simulink library "simulink"  (R2014a)
settings: Solver=ode45  SolverMode=SingleTasking  StartTime=0.0  StopTime=10.0  RelTol=1e-3
PostLoadFcn:
  | setsysloc_simulink(bdroot)
undefined symbols (not defined in the file or in its folder): DiscIntNeverNeededParam, getdatatypespecs, NumBits1, NumBits2, sfunxy, sigbuilder_block, slcm, SlDemoSign, Slope1, Slope2
libraries: simulink x40, sl_helperblocks x2, eml_lib x1
(part 5 of 5)

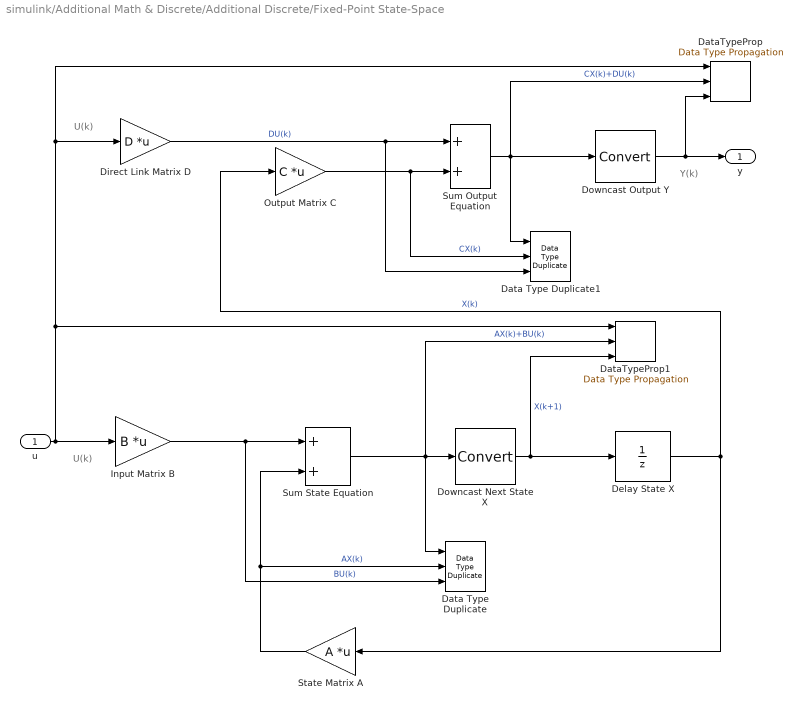
== system simulink/Additional Math & Discrete/Additional Discrete/Fixed-Point State-Space ==
  note: U(k)
  note: U(k)
  note: Y(k)
  u : Inport
  Data Type Duplicate : DataTypeDuplicate  DisableCoverage=on  NumInputPorts=3
  Data Type Duplicate1 : DataTypeDuplicate  DisableCoverage=on  NumInputPorts=3
  DataTypeProp : simulink/Signal Attributes/Data Type Propagation  PropDataType=fixdt(1, 16)  IfRefDouble=double  IfRefSingle=single  IsSigned=IsSigned1 or IsSigned2  NumBitsBase=NumBits1  NumBitsMult=1  NumBitsAdd=0  NumBitsAllowFinal=1:128  PropScaling=2^-10  ValuesUsedBestPrec=[5 -7]  SlopeBase=PosRange2  SlopeMult=1  SlopeAdd=0  BiasBase=Bias2  BiasMult=1  BiasAdd=0
  DataTypeProp1 : simulink/Signal Attributes/Data Type Propagation  PropDataType=fixdt(1, 16)  IfRefDouble=double  IfRefSingle=single  IsSigned=IsSigned1 or IsSigned2  NumBitsBase=NumBits1  NumBitsMult=1  NumBitsAdd=0  NumBitsAllowFinal=1:128  PropScaling=2^-10  ValuesUsedBestPrec=[5 -7]  SlopeBase=PosRange2  SlopeMult=1  SlopeAdd=0  BiasBase=Bias2  BiasMult=1  BiasAdd=0
  Delay State X : UnitDelay  Description=Store in Global RAM  DisableCoverage=on  InitialCondition=X0  SampleTime=-1
      settings: AttributesFormatString=%<Description>
  Direct Link Matrix D : Gain  Description=Multiply in CPU  DisableCoverage=on  Gain=D  Multiplication=Matrix(K*u) (u vector)  OutDataTypeStr=Inherit: Inherit via back propagation
      settings: AttributesFormatString=%<Description>
  Downcast Next State X : DataTypeConversion  Description=|  DisableCoverage=on
      | Reduce from CPU Size
      |  to Global RAM Size
      settings: AttributesFormatString=%<Description>
  Downcast Output Y : DataTypeConversion  Description=|
      | Reduce from CPU Size
      |  to Global RAM Size
      settings: AttributesFormatString=%<Description>
  Input Matrix B : Gain  Description=Multiply in CPU  DisableCoverage=on  Gain=B  Multiplication=Matrix(K*u) (u vector)  OutDataTypeStr=Inherit: Inherit via back propagation
      settings: AttributesFormatString=%<Description>
  Output Matrix C : Gain  Description=Multiply in CPU  DisableCoverage=on  Gain=C  Multiplication=Matrix(K*u) (u vector)  OutDataTypeStr=Inherit: Inherit via back propagation
      settings: AttributesFormatString=%<Description>
  State Matrix A : Gain  Description=Multiply in CPU  DisableCoverage=on  Gain=A  Multiplication=Matrix(K*u) (u vector)  OutDataTypeStr=Inherit: Inherit via back propagation
      settings: AttributesFormatString=%<Description>
  Sum Output Equation : Sum  Description=Add in CPU  DisableCoverage=on  OutDataTypeStr=slDataTypeAndScale(('InternalDataType'),('OutputEqScaling'))
      settings: AttributesFormatString=%<Description>
  Sum State Equation : Sum  Description=Add in CPU  DisableCoverage=on  OutDataTypeStr=slDataTypeAndScale(('InternalDataType'),('StateEqScaling'))
      settings: AttributesFormatString=%<Description>
  y : Outport  InitialOutput=0
  wires:
  Direct Link Matrix D/1 -> Data Type Duplicate1/3, Sum Output Equation/1  "DU(k)"
  Output Matrix C/1 -> Data Type Duplicate1/2, Sum Output Equation/2  "CX(k)"
  Sum Output Equation/1 -> DataTypeProp/2, Data Type Duplicate1/1, Downcast Output Y/1  "CX(k)+DU(k)"
  Downcast Output Y/1 -> DataTypeProp/3, y/1
  Delay State X/1 -> Output Matrix C/1, State Matrix A/1  "X(k)"
  Downcast Next State X/1 -> DataTypeProp1/3, Delay State X/1  "X(k+1)"
  Sum State Equation/1 -> DataTypeProp1/2, Data Type Duplicate/1, Downcast Next State X/1  "AX(k)+BU(k)"
  Input Matrix B/1 -> Data Type Duplicate/3, Sum State Equation/1  "BU(k)"
  u/1 -> DataTypeProp1/1, DataTypeProp/1, Direct Link Matrix D/1, Input Matrix B/1
  State Matrix A/1 -> Data Type Duplicate/2, Sum State Equation/2  "AX(k)"

== system simulink/Additional Math & Discrete/Additional Discrete/Transfer Fcn Direct Form II ==
  u : Inport
  DataTypeProp : simulink/Signal Attributes/Data Type Propagation  PropDataType=fixdt(1, 16)  IfRefDouble=double  IfRefSingle=single  IsSigned=IsSigned1 or IsSigned2  NumBitsBase=max([NumBits1 NumBits2])  NumBitsMult=1  NumBitsAdd=0  NumBitsAllowFinal=1:128  PropScaling=2^-10  ValuesUsedBestPrec=[5 -7]  SlopeBase=min([Slope1 Slope2])  SlopeMult=OutputSlopeMult  SlopeAdd=0  BiasBase=Bias1  BiasMult=0  BiasAdd=0
  DataTypeProp1 : simulink/Signal Attributes/Data Type Propagation  PropDataType=fixdt(1, 16)  IfRefDouble=double  IfRefSingle=single  IsSigned=IsSigned1 or IsSigned2  NumBitsBase=max([NumBits1 NumBits2])  NumBitsMult=1  NumBitsAdd=0  NumBitsAllowFinal=1:128  PropScaling=2^-10  ValuesUsedBestPrec=[5 -7]  SlopeBase=min([Slope1 Slope2])  SlopeMult=OutputSlopeMult2  SlopeAdd=0  BiasBase=Bias1  BiasMult=0  BiasAdd=0
  DenCoef : Gain  DisableCoverage=on  Gain=DenCoefVec  Multiplication=Matrix(K*u) (u vector)
      settings: AttributesFormatString=|
      | Data Type and Scaling Inherited
      | with goal of NO Quantization Noise
      | Possible Overflow or Saturation
  Downcast : DataTypeConversion  Description=|  LockScale=on
      | Reduce from CPU Size
      |  to Global RAM Size
      settings: AttributesFormatString=%<Description>
  Downcast1 : DataTypeConversion  Description=|  DisableCoverage=on  LockScale=on
      | Reduce from CPU Size
      |  to Global RAM Size
      settings: AttributesFormatString=%<Description>
  Mux : Mux  Inputs=2
  NumCoef : Gain  DisableCoverage=on  Gain=NumCoefVec  Multiplication=Matrix(K*u) (u vector)
      settings: AttributesFormatString=|
      | Data Type and Scaling Inherited
      | with goal of NO Quantization Noise
      | Possible Overflow or Saturation
  Sum : Sum  Tag=S16 2^-10  DisableCoverage=on  Inputs=+-  LockScale=on
      settings: AttributesFormatString=|
      | Data Type and Scaling Inherited
      | with goal of NO Quantization Noise
      | Possible Overflow or Saturation
  Tapped Delay : simulink/Discrete/Tapped Delay  vinit=vinit  samptime=-1  NumDelays=-1  DelayOrder=Newest  includeCurrent=off
      settings: AttributesFormatString=|
      | Number of Taps
      | Inherited via Back Propagation
  y : Outport
  wires:
  Sum/1 -> Downcast1/1
  DenCoef/1 -> Sum/2
  u/1 -> DataTypeProp1/1, DataTypeProp1/2, DataTypeProp/2, DataTypeProp/1, Sum/1
  NumCoef/1 -> Downcast/1
  Tapped Delay/1 -> DenCoef/1, Mux/2
  Downcast1/1 -> DataTypeProp1/3, Mux/1, Tapped Delay/1
  Mux/1 -> NumCoef/1
  Downcast/1 -> y/1, DataTypeProp/3

== system simulink/Additional Math & Discrete/Additional Discrete/Transfer Fcn Direct Form II Time Varying ==
  u : Inport
  Num : Inport  Port=2
  Den No Lead : Inport  Port=3
  DataTypeProp : simulink/Signal Attributes/Data Type Propagation  PropDataType=fixdt(1, 16)  IfRefDouble=double  IfRefSingle=single  IsSigned=IsSigned1  NumBitsBase=NumBits1  NumBitsMult=1  NumBitsAdd=0  NumBitsAllowFinal=1:128  PropScaling=2^-10  ValuesUsedBestPrec=[5 -7]  SlopeBase=Slope1  SlopeMult=1  SlopeAdd=0  BiasBase=Bias1  BiasMult=1  BiasAdd=0
  DataTypeProp1 : simulink/Signal Attributes/Data Type Propagation  PropDataType=fixdt(1, 16)  IfRefDouble=double  IfRefSingle=single  IsSigned=IsSigned1  NumBitsBase=NumBits1  NumBitsMult=1  NumBitsAdd=0  NumBitsAllowFinal=1:128  PropScaling=2^-10  ValuesUsedBestPrec=[5 -7]  SlopeBase=Slope1  SlopeMult=2  SlopeAdd=0  BiasBase=Bias1  BiasMult=1  BiasAdd=0
  Dot1 : DotProduct  DisableCoverage=on  OutDataTypeStr=Inherit: Inherit via internal rule
      settings: AttributesFormatString=|
      | Data Type and Scaling Inherited
      | with goal of NO Quantization Noise
      | Possible Overflow or Saturation
  Dot2 : DotProduct  DisableCoverage=on  OutDataTypeStr=Inherit: Inherit via internal rule
      settings: AttributesFormatString=|
      | Data Type and Scaling Inherited
      | with goal of NO Quantization Noise
      | Possible Overflow or Saturation
  Downcast : DataTypeConversion  Description=|  LockScale=on
      | Reduce from CPU Size
      |  to Global RAM Size
      settings: AttributesFormatString=%<Description>
  Downcast1 : DataTypeConversion  Description=|  DisableCoverage=on  LockScale=on
      | Reduce from CPU Size
      |  to Global RAM Size
      settings: AttributesFormatString=%<Description>
  Mux : Mux  Inputs=2
  Sum : Sum  Tag=S16 2^-10  DisableCoverage=on  Inputs=+-  LockScale=on
      settings: AttributesFormatString=|
      | Data Type and Scaling Inherited
      | with goal of NO Quantization Noise
      | Possible Overflow or Saturation
  Tapped Delay : simulink/Discrete/Tapped Delay  vinit=vinit  samptime=-1  NumDelays=-1  DelayOrder=Newest  includeCurrent=off
      settings: AttributesFormatString=|
      | Number of Taps
      | Inherited via Back Propagation
  y : Outport
  wires:
  Den No Lead/1 -> Dot1/2
  Num/1 -> Dot2/2
  Downcast/1 -> DataTypeProp/3, y/1
  Mux/1 -> Dot2/1
  Downcast1/1 -> DataTypeProp1/3, Tapped Delay/1, Mux/1
  Tapped Delay/1 -> Dot1/1, Mux/2
  Dot2/1 -> Downcast/1
  u/1 -> Sum/1, DataTypeProp1/2, DataTypeProp1/1, DataTypeProp/2, DataTypeProp/1
  Dot1/1 -> Sum/2
  Sum/1 -> Downcast1/1

== system simulink/Additional Math & Discrete/Additional Discrete/Unit Delay Enabled ==
  note: Enable
  note: Xold
  u : Inport
  E : Inport  Port=2
  Enable : Switch  Criteria=u2 ~= 0  OutDataTypeStr=Inherit: Inherit via back propagation  ZeroCross=off
  FixPt Data Type Duplicate1 : DataTypeDuplicate  DisableCoverage=on  NumInputPorts=3
  FixPt Unit Delay1 : UnitDelay  InitialCondition=vinit  SampleTime=tsamp  HasFrameUpgradeWarning=off
  y : Outport
  wires:
  E/1 -> Enable/2
  u/1 -> FixPt Data Type Duplicate1/3, Enable/1
  Enable/1 -> FixPt Unit Delay1/1, FixPt Data Type Duplicate1/2  "Xnew"
  FixPt Unit Delay1/1 -> y/1, Enable/3, FixPt Data Type Duplicate1/1

== system simulink/Additional Math & Discrete/Additional Discrete/Unit Delay Enabled External IC ==
  note: Enable
  note: Initial Value
  u : Inport
  E : Inport  Port=2
  IC : Inport  Port=3
  Enable : Switch  Criteria=u2 ~= 0  OutDataTypeStr=Inherit: Inherit via back propagation  ZeroCross=off
  FixPt Data Type Duplicate1 : DataTypeDuplicate  DisableCoverage=on  NumInputPorts=4
  Unit Delay External IC : simulink/Additional Math & Discrete/Additional Discrete/Unit Delay External IC  tsamp=tsamp
  y : Outport
  wires:
  E/1 -> Enable/2
  IC/1 -> FixPt Data Type Duplicate1/3, Unit Delay External IC/2
  u/1 -> FixPt Data Type Duplicate1/4, Enable/1
  Enable/1 -> FixPt Data Type Duplicate1/2, Unit Delay External IC/1  "Xnew"
  Unit Delay External IC/1 -> y/1, Enable/3, FixPt Data Type Duplicate1/1

== system simulink/Additional Math & Discrete/Additional Discrete/Unit Delay Enabled Resettable ==
  note: Enable
  note: Reset
  u : Inport
  E : Inport  Port=2
  R : Inport  Port=3
  Enable : Switch  Criteria=u2 ~= 0  OutDataTypeStr=Inherit: Inherit via back propagation  ZeroCross=off
  FixPt Data Type Duplicate2 : DataTypeDuplicate  DisableCoverage=on  NumInputPorts=3
  Unit Delay Resettable : simulink/Additional Math & Discrete/Additional Discrete/Unit Delay Resettable  vinit=vinit  tsamp=tsamp
  y : Outport
  wires:
  E/1 -> Enable/2
  u/1 -> Enable/1, FixPt Data Type Duplicate2/3
  Enable/1 -> FixPt Data Type Duplicate2/2, Unit Delay Resettable/1  "Xnew"
  Unit Delay Resettable/1 -> FixPt Data Type Duplicate2/1, Enable/3, y/1
  R/1 -> Unit Delay Resettable/2

== system simulink/Additional Math & Discrete/Additional Discrete/Unit Delay Enabled Resettable External IC ==
  note: Enable
  note: Reset
  note: Initial Value
  u : Inport
  E : Inport  Port=2
  R : Inport  Port=3
  IC : Inport  Port=4
  Enable : Switch  Criteria=u2 ~= 0  OutDataTypeStr=Inherit: Inherit via back propagation  ZeroCross=off
  FixPt Data Type Duplicate1 : DataTypeDuplicate  DisableCoverage=on  NumInputPorts=4
  Unit Delay Resettable External IC : simulink/Additional Math & Discrete/Additional Discrete/Unit Delay Resettable External IC  tsamp=tsamp
  y : Outport
  wires:
  Unit Delay Resettable External IC/1 -> y/1, Enable/3, FixPt Data Type Duplicate1/1
  R/1 -> Unit Delay Resettable External IC/2
  Enable/1 -> Unit Delay Resettable External IC/1, FixPt Data Type Duplicate1/3
  u/1 -> Enable/1, FixPt Data Type Duplicate1/4
  IC/1 -> Unit Delay Resettable External IC/3, FixPt Data Type Duplicate1/2
  E/1 -> Enable/2

== system simulink/Additional Math & Discrete/Additional Discrete/Unit Delay External IC ==
  note: Xnew
  note: Initial Value
  u : Inport
  IC : Inport  Port=2
  FixPt Constant : Constant  DisableCoverage=on  Value=0  OutDataTypeStr=fixdt(0,8,0)
  FixPt Data Type Duplicate1 : DataTypeDuplicate  DisableCoverage=on  NumInputPorts=3
  FixPt Unit Delay1 : UnitDelay  DisableCoverage=on  InitialCondition=0.0  SampleTime=tsamp  HasFrameUpgradeWarning=off
  FixPt Unit Delay2 : UnitDelay  DisableCoverage=on  InitialCondition=1  SampleTime=tsamp
  Init : Switch  Criteria=u2 ~= 0  OutDataTypeStr=Inherit: Inherit via back propagation  ZeroCross=off
  y : Outport
  wires:
  FixPt Unit Delay1/1 -> Init/3  "Xold"
  Init/1 -> y/1, FixPt Data Type Duplicate1/1
  FixPt Unit Delay2/1 -> Init/2
  FixPt Constant/1 -> FixPt Unit Delay2/1
  u/1 -> FixPt Unit Delay1/1, FixPt Data Type Duplicate1/2
  IC/1 -> Init/1, FixPt Data Type Duplicate1/3

== system simulink/Additional Math & Discrete/Additional Discrete/Unit Delay Resettable ==
  note: Reset
  u : Inport
  R : Inport  Port=2
  FixPt Constant : Constant  DisableCoverage=on  Value=0  OutDataTypeStr=fixdt(0,8,0)
  FixPt Data Type Duplicate1 : DataTypeDuplicate  DisableCoverage=on  NumInputPorts=4
  FixPt Logical Operator : Logic  DisableCoverage=on  Operator=OR  AllPortsSameDT=off  OutDataTypeStr=fixdt(0, 8)
  FixPt Unit Delay1 : UnitDelay  DisableCoverage=on  InitialCondition=vinit  SampleTime=tsamp  HasFrameUpgradeWarning=off
  FixPt Unit Delay2 : UnitDelay  DisableCoverage=on  InitialCondition=1  SampleTime=tsamp
  Init : Switch  Criteria=u2 ~= 0  OutDataTypeStr=Inherit: Inherit via back propagation  ZeroCross=off
  Initial Condition : Constant  DisableCoverage=on  Value=vinit  OutDataTypeStr=Inherit: Inherit via back propagation
  Reset : Switch  Criteria=u2 ~= 0  OutDataTypeStr=Inherit: Inherit via back propagation  ZeroCross=off
  y : Outport
  wires:
  Initial Condition/1 -> Reset/1, Init/1, FixPt Data Type Duplicate1/3  "Initial Value"
  u/1 -> FixPt Data Type Duplicate1/4, Reset/3
  Reset/1 -> FixPt Data Type Duplicate1/2, FixPt Unit Delay1/1  "Xnew"
  R/1 -> Reset/2, FixPt Logical Operator/1
  FixPt Constant/1 -> FixPt Unit Delay2/1
  FixPt Unit Delay2/1 -> FixPt Logical Operator/2
  Init/1 -> FixPt Data Type Duplicate1/1, y/1
  FixPt Unit Delay1/1 -> Init/3  "Xold"
  FixPt Logical Operator/1 -> Init/2

== system simulink/Additional Math & Discrete/Additional Discrete/Unit Delay Resettable External IC ==
  note: Initial Value
  note: Reset
  u : Inport
  R : Inport  Port=2
  IC : Inport  Port=3
  FixPt Constant : Constant  DisableCoverage=on  Value=0  OutDataTypeStr=fixdt(0,8,0)
  FixPt Data Type Duplicate1 : DataTypeDuplicate  DisableCoverage=on  NumInputPorts=4
  FixPt Logical Operator : Logic  DisableCoverage=on  Operator=OR  AllPortsSameDT=off  OutDataTypeStr=fixdt(0, 8)
  FixPt Unit Delay1 : UnitDelay  DisableCoverage=on  InitialCondition=0.0  SampleTime=tsamp  HasFrameUpgradeWarning=off
  FixPt Unit Delay2 : UnitDelay  DisableCoverage=on  InitialCondition=1  SampleTime=tsamp
  Init : Switch  Criteria=u2 ~= 0  OutDataTypeStr=Inherit: Inherit via back propagation  ZeroCross=off
  Reset : Switch  Criteria=u2 ~= 0  OutDataTypeStr=Inherit: Inherit via back propagation  ZeroCross=off
  y : Outport
  wires:
  IC/1 -> Reset/1, Init/1, FixPt Data Type Duplicate1/3
  u/1 -> FixPt Data Type Duplicate1/4, Reset/3
  Reset/1 -> FixPt Data Type Duplicate1/2, FixPt Unit Delay1/1  "Xnew"
  R/1 -> Reset/2, FixPt Logical Operator/1
  FixPt Constant/1 -> FixPt Unit Delay2/1
  FixPt Unit Delay2/1 -> FixPt Logical Operator/2
  Init/1 -> FixPt Data Type Duplicate1/1, y/1
  FixPt Unit Delay1/1 -> Init/3  "Xold"
  FixPt Logical Operator/1 -> Init/2

== system simulink/Additional Math & Discrete/Additional Discrete/Unit Delay With Preview Enabled ==
  note: Enable
  note: Xnew
  note: Xnew
  note: Xold
  u : Inport
  E : Inport  Port=2
  Enable : Switch  Criteria=u2 ~= 0  OutDataTypeStr=Inherit: Inherit via back propagation  ZeroCross=off
  FixPt Data Type Duplicate1 : DataTypeDuplicate  DisableCoverage=on  NumInputPorts=3
  FixPt Unit Delay1 : UnitDelay  InitialCondition=vinit  SampleTime=tsamp  HasFrameUpgradeWarning=off
  y : Outport
  x : Outport  Port=2
  wires:
  FixPt Unit Delay1/1 -> FixPt Data Type Duplicate1/1, Enable/3, x/1
  Enable/1 -> FixPt Data Type Duplicate1/2, FixPt Unit Delay1/1, y/1
  u/1 -> Enable/1, FixPt Data Type Duplicate1/3
  E/1 -> Enable/2

== system simulink/Additional Math & Discrete/Additional Discrete/Unit Delay With Preview Enabled Resettable ==
  note: Enable
  note: Xold
  note: Xnew
  note: Reset
  u : Inport
  E : Inport  Port=2
  R : Inport  Port=3
  Enable : Switch  Criteria=u2 ~= 0  OutDataTypeStr=Inherit: Inherit via back propagation  ZeroCross=off
  FixPt Data Type Duplicate2 : DataTypeDuplicate  DisableCoverage=on  NumInputPorts=5
  FixPt Unit Delay1 : UnitDelay  InitialCondition=vinit  SampleTime=tsamp  HasFrameUpgradeWarning=off
  Initial Condition : Constant  DisableCoverage=on  Value=vinit  OutDataTypeStr=Inherit: Inherit via back propagation
  Reset : Switch  Criteria=u2 ~= 0  OutDataTypeStr=Inherit: Inherit via back propagation  InputSameDT=on
  y : Outport
  x : Outport  Port=2
  wires:
  E/1 -> Enable/2
  Initial Condition/1 -> FixPt Data Type Duplicate2/3, Reset/1  "Reset Value"
  u/1 -> FixPt Data Type Duplicate2/5, Enable/1
  Enable/1 -> FixPt Data Type Duplicate2/4, Reset/3
  FixPt Unit Delay1/1 -> x/1, Enable/3, FixPt Data Type Duplicate2/1
  Reset/1 -> y/1, FixPt Data Type Duplicate2/2, FixPt Unit Delay1/1
  R/1 -> Reset/2

== system simulink/Additional Math & Discrete/Additional Discrete/Unit Delay With Preview Enabled Resettable External RV ==
  note: Enable
  note: Input
  note: Reset
  note: Reset Value
  note: Xnew
  note: Xold
  u : Inport
  E : Inport  Port=2
  R : Inport  Port=3
  V : Inport  Port=4
  Enable : Switch  Criteria=u2 ~= 0  OutDataTypeStr=Inherit: Inherit via back propagation  ZeroCross=off
  FixPt Data Type Duplicate2 : DataTypeDuplicate  DisableCoverage=on  NumInputPorts=5
  FixPt Unit Delay1 : UnitDelay  InitialCondition=vinit  SampleTime=tsamp  HasFrameUpgradeWarning=off
  Reset : Switch  Criteria=u2 ~= 0  OutDataTypeStr=Inherit: Inherit via back propagation  InputSameDT=on
  y1 : Outport
  y2 : Outport  Port=2
  wires:
  R/1 -> Reset/2
  Reset/1 -> FixPt Unit Delay1/1, FixPt Data Type Duplicate2/2, y1/1
  FixPt Unit Delay1/1 -> FixPt Data Type Duplicate2/1, Enable/3, y2/1
  Enable/1 -> Reset/3, FixPt Data Type Duplicate2/4
  u/1 -> Enable/1, FixPt Data Type Duplicate2/5
  V/1 -> Reset/1, FixPt Data Type Duplicate2/3
  E/1 -> Enable/2

== system simulink/Additional Math & Discrete/Additional Discrete/Unit Delay With Preview Resettable ==
  note: Reset
  note: Xnew
  note: Xold
  u : Inport
  R : Inport  Port=2
  FixPt Data Type Duplicate2 : DataTypeDuplicate  DisableCoverage=on  NumInputPorts=4
  FixPt Unit Delay1 : UnitDelay  InitialCondition=vinit  SampleTime=tsamp  HasFrameUpgradeWarning=off
  Initial Condition : Constant  DisableCoverage=on  Value=vinit  OutDataTypeStr=Inherit: Inherit via back propagation
  Reset : Switch  Criteria=u2 ~= 0  OutDataTypeStr=Inherit: Inherit via back propagation  ZeroCross=off
  y : Outport
  x : Outport  Port=2
  wires:
  Initial Condition/1 -> FixPt Data Type Duplicate2/3, Reset/1  "Reset Value"
  u/1 -> Reset/3, FixPt Data Type Duplicate2/4
  FixPt Unit Delay1/1 -> x/1, FixPt Data Type Duplicate2/1
  Reset/1 -> y/1, FixPt Data Type Duplicate2/2, FixPt Unit Delay1/1
  R/1 -> Reset/2

== system simulink/Additional Math & Discrete/Additional Discrete/Unit Delay With Preview Resettable External RV ==
  note: Reset Value
  note: Reset
  note: Xnew
  note: Xold
  u : Inport
  R : Inport  Port=2
  RV : Inport  Port=3
  FixPt Data Type Duplicate2 : DataTypeDuplicate  DisableCoverage=on  NumInputPorts=4
  FixPt Unit Delay1 : UnitDelay  InitialCondition=vinit  SampleTime=tsamp  HasFrameUpgradeWarning=off
  Reset : Switch  Criteria=u2 ~= 0  OutDataTypeStr=Inherit: Inherit via back propagation  ZeroCross=off
  y : Outport
  x : Outport  Port=2
  wires:
  RV/1 -> FixPt Data Type Duplicate2/3, Reset/1
  FixPt Unit Delay1/1 -> x/1, FixPt Data Type Duplicate2/1
  Reset/1 -> y/1, FixPt Data Type Duplicate2/2, FixPt Unit Delay1/1
  R/1 -> Reset/2
  u/1 -> Reset/3, FixPt Data Type Duplicate2/4

== system simulink/Additional Math & Discrete/Additional Math: Increment - Decrement/Decrement Real World ==
  u : Inport
  FixPt Constant : Constant  DisableCoverage=on  OutDataTypeStr=Inherit: Inherit via back propagation
  FixPt Data Type Duplicate : DataTypeDuplicate  DisableCoverage=on  NumInputPorts=3
  FixPt Sum1 : Sum  Inputs=+-  OutDataTypeStr=Inherit: Inherit via back propagation  InputSameDT=on  LockScale=on
  y : Outport
  wires:
  FixPt Sum1/1 -> y/1, FixPt Data Type Duplicate/1
  FixPt Constant/1 -> FixPt Sum1/2, FixPt Data Type Duplicate/3
  u/1 -> FixPt Sum1/1, FixPt Data Type Duplicate/2

== system simulink/Additional Math & Discrete/Additional Math: Increment - Decrement/Decrement Stored Integer ==
  u : Inport
  FixPt Constant : Constant  DisableCoverage=on  OutDataTypeStr=Inherit: Inherit via back propagation
  FixPt Data Type Duplicate : DataTypeDuplicate  DisableCoverage=on  NumInputPorts=3
  FixPt Data Type Propagation : simulink/Signal Attributes/Data Type Propagation  PropDataType=fixdt(1, 16)  IfRefDouble=double  IfRefSingle=single  IsSigned=IsSigned1  NumBitsBase=NumBits1  NumBitsMult=1  NumBitsAdd=0  NumBitsAllowFinal=1:128  PropScaling=2^-10  ValuesUsedBestPrec=[5 -7]  SlopeBase=Slope1  SlopeMult=0  SlopeAdd=1  BiasBase=Bias1  BiasMult=0  BiasAdd=0
  FixPt Gateway In : DataTypeConversion  DisableCoverage=on  ConvertRealWorld=Stored Integer (SI)
  FixPt Sum1 : Sum  Inputs=+-  OutDataTypeStr=Inherit: Inherit via back propagation  InputSameDT=on  LockScale=on
  y : Outport
  wires:
  u/1 -> FixPt Data Type Duplicate/2, FixPt Sum1/1
  FixPt Constant/1 -> FixPt Gateway In/1, FixPt Data Type Propagation/3
  FixPt Sum1/1 -> FixPt Data Type Duplicate/1, y/1
  FixPt Gateway In/1 -> FixPt Data Type Duplicate/3, FixPt Sum1/2, FixPt Data Type Propagation/1, FixPt Data Type Propagation/2

== system simulink/Additional Math & Discrete/Additional Math: Increment - Decrement/Decrement To Zero ==
  u : Inport
  FixPt Constant : Constant  DisableCoverage=on  OutDataTypeStr=Inherit: Inherit via back propagation
  FixPt Data Type Duplicate : DataTypeDuplicate  DisableCoverage=on  NumInputPorts=5
  FixPt Relational Operator3 : RelationalOperator  DisableCoverage=on  Operator=>  OutDataTypeStr=boolean  ZeroCross=off
  FixPt Sum1 : Sum  DisableCoverage=on  Inputs=+-  OutDataTypeStr=Inherit: Inherit via back propagation  LockScale=on
  FixPt Switch4 : Switch  Criteria=u2 ~= 0  Threshold=1  OutDataTypeStr=Inherit: Inherit via back propagation  ZeroCross=off
  Ground1 : Ground  DisableCoverage=on
  y : Outport
  wires:
  FixPt Switch4/1 -> FixPt Data Type Duplicate/1, y/1
  Ground1/1 -> FixPt Data Type Duplicate/2, FixPt Switch4/3
  FixPt Relational Operator3/1 -> FixPt Switch4/2
  u/1 -> FixPt Relational Operator3/1, FixPt Data Type Duplicate/4, FixPt Sum1/1
  FixPt Constant/1 -> FixPt Relational Operator3/2, FixPt Data Type Duplicate/5, FixPt Sum1/2
  FixPt Sum1/1 -> FixPt Switch4/1, FixPt Data Type Duplicate/3

== system simulink/Additional Math & Discrete/Additional Math: Increment - Decrement/Decrement Time To Zero ==
  u : Inport
  FixPt Data Type Duplicate : DataTypeDuplicate  DisableCoverage=on  NumInputPorts=5
  FixPt Relational Operator3 : RelationalOperator  DisableCoverage=on  Operator=>  OutDataTypeStr=boolean  ZeroCross=off
  FixPt Sample Time Math : SampleTimeMath  DisableCoverage=on  TsampMathOp=Ts Only  OutDataTypeStr=Inherit: Inherit via back propagation
  FixPt Sum1 : Sum  DisableCoverage=on  Inputs=+-  OutDataTypeStr=Inherit: Inherit via back propagation  LockScale=on
  FixPt Switch4 : Switch  Criteria=u2 ~= 0  Threshold=1  OutDataTypeStr=Inherit: Inherit via back propagation  ZeroCross=off
  Ground1 : Ground  DisableCoverage=on
  y : Outport
  wires:
  FixPt Switch4/1 -> FixPt Data Type Duplicate/1, y/1
  Ground1/1 -> FixPt Data Type Duplicate/2, FixPt Switch4/3
  FixPt Relational Operator3/1 -> FixPt Switch4/2
  u/1 -> FixPt Relational Operator3/1, FixPt Data Type Duplicate/4, FixPt Sum1/1, FixPt Sample Time Math/1
  FixPt Sample Time Math/1 -> FixPt Relational Operator3/2, FixPt Data Type Duplicate/5, FixPt Sum1/2
  FixPt Sum1/1 -> FixPt Switch4/1, FixPt Data Type Duplicate/3

== system simulink/Additional Math & Discrete/Additional Math: Increment - Decrement/Increment Real World ==
  u : Inport
  FixPt Constant : Constant  DisableCoverage=on  OutDataTypeStr=Inherit: Inherit via back propagation
  FixPt Data Type Duplicate : DataTypeDuplicate  DisableCoverage=on  NumInputPorts=3
  FixPt Sum1 : Sum  OutDataTypeStr=Inherit: Inherit via back propagation  InputSameDT=on  LockScale=on
  y : Outport
  wires:
  u/1 -> FixPt Data Type Duplicate/2, FixPt Sum1/1
  FixPt Constant/1 -> FixPt Data Type Duplicate/3, FixPt Sum1/2
  FixPt Sum1/1 -> FixPt Data Type Duplicate/1, y/1

== system simulink/Additional Math & Discrete/Additional Math: Increment - Decrement/Increment Stored Integer ==
  u : Inport
  FixPt Constant : Constant  DisableCoverage=on  OutDataTypeStr=Inherit: Inherit via back propagation
  FixPt Data Type Duplicate : DataTypeDuplicate  DisableCoverage=on  NumInputPorts=3
  FixPt Data Type Propagation : simulink/Signal Attributes/Data Type Propagation  PropDataType=fixdt(1, 16)  IfRefDouble=double  IfRefSingle=single  IsSigned=IsSigned1  NumBitsBase=NumBits1  NumBitsMult=1  NumBitsAdd=0  NumBitsAllowFinal=1:128  PropScaling=2^-10  ValuesUsedBestPrec=[5 -7]  SlopeBase=Slope1  SlopeMult=0  SlopeAdd=1  BiasBase=Bias1  BiasMult=0  BiasAdd=0
  FixPt Gateway In : DataTypeConversion  DisableCoverage=on  ConvertRealWorld=Stored Integer (SI)
  FixPt Sum1 : Sum  OutDataTypeStr=Inherit: Inherit via back propagation  InputSameDT=on  LockScale=on
  y : Outport
  wires:
  FixPt Gateway In/1 -> FixPt Data Type Propagation/2, FixPt Data Type Propagation/1, FixPt Sum1/2, FixPt Data Type Duplicate/3
  FixPt Sum1/1 -> y/1, FixPt Data Type Duplicate/1
  FixPt Constant/1 -> FixPt Data Type Propagation/3, FixPt Gateway In/1
  u/1 -> FixPt Sum1/1, FixPt Data Type Duplicate/2

== system simulink/Model Verification/Check Input Resolution/fixed ==
  u : Inport
  resolution : Inport  Port=2
  fold : Logic  DisableCoverage=on  Operator=OR  Inputs=1
  relop : RelationalOperator  DisableCoverage=on  Operator===  InputSameDT=on
  out : Outport
  wires:
  u/1 -> relop/1
  resolution/1 -> relop/2
  relop/1 -> fold/1
  fold/1 -> out/1

== system simulink/Model Verification/Check Input Resolution/steps ==
  u : Inport
  resolution : Inport  Port=2
  relop : RelationalOperator  DisableCoverage=on  Operator=<=  InputSameDT=on
  rem : Math  DisableCoverage=on  Operator=mod  SaturateOnIntegerOverflow=on
  tol : Constant  DisableCoverage=on  Value=10e-3
  out : Outport
  wires:
  u/1 -> rem/1
  resolution/1 -> rem/2
  rem/1 -> relop/1
  tol/1 -> relop/2
  relop/1 -> out/1

== system simulink/Model-Wide Utilities/Block Support Table/EmptySubsystem ==

== system simulink/Model-Wide Utilities/DocBlock/EmptySubsystem ==

== system simulink/Model-Wide Utilities/Model Info/EmptySubsystem ==

== system simulink/Model-Wide Utilities/Timed-Based Linearization/Triggered Linearization ==
  Trigger : TriggerPort
  MATLAB S-Function : M-S-Function  DisableCoverage=on  FunctionName=sfunlin  Parameters=name_,SampleTime
